simulink subsystem "plant"  (R2020b)
settings: Solver=VariableStepAuto  StartTime=0.0  StopTime=10.0  RelTol=1e-3
settings Model: Creator=leop9  LastModifiedBy=Previ

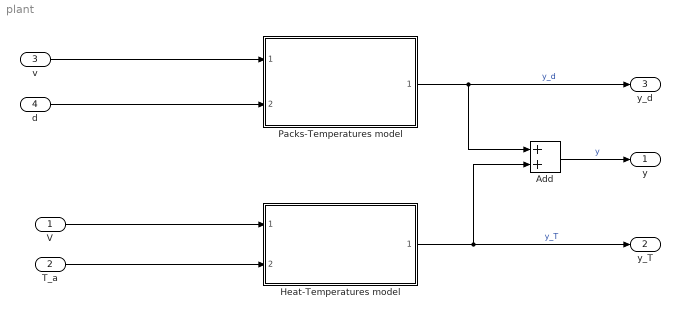
== system plant ==
  V : Inport
  T_a : Inport  Port=2
  v : Inport  Port=3
  d : Inport  Port=4
  Add : Sum
  Heat-Temperatures model : Subsystem  ReferencedSubsystem=heat_temperatures_12
  Packs-Temperatures model : Subsystem  ReferencedSubsystem=packs_temperatures_12
  y : Outport
  y_T : Outport  Port=2
  y_d : Outport  Port=3
  wires:
  v/1 -> Packs-Temperatures model/1
  d/1 -> Packs-Temperatures model/2
  V/1 -> Heat-Temperatures model/1
  T_a/1 -> Heat-Temperatures model/2
  Packs-Temperatures model/1 -> Add/1, y_d/1  "y_d"
  Heat-Temperatures model/1 -> Add/2, y_T/1  "y_T"
  Add/1 -> y/1  "y"
